simulink model "Controller"  (R2014a)
settings: Solver=FixedStepDiscrete  StartTime=0.0  StopTime=100  FixedStep=0.001  MaxStep=0.01  RelTol=1e-4
InitFcn:
  | Mot_Init
undefined symbols (not defined in the file): Actuator_Length, ControllerRate, Dig_Limit, LowerProtectionFraction, Ratio, SampleSize, UpperProtectionFraction
libraries: simulink x8
settings Model: DSRTSU_INTERNAL_RTI_VER=460  DSRTSU_INTERNAL_RTI_TYPE=rti1006  CovModelRefEnable=off  Creator=jstoddar  LastModifiedBy=uaEcoCar3
settings DataIOCC: SaveFormat=StructureWithTime  SaveOutput=off  SaveTime=off
settings OptimizationCC: ExpressionDepthLimit=2147483647  LifeSpan=1
settings DebuggingCC: UnderspecifiedInitializationDetection=Classic  SolverPrmCheckMsg=none  FcnCallInpInsideContextMsg=EnableAllAsWarning  FrameProcessingCompatibilityMsg=error  StateNameClashWarn=warning
settings HardwareCC: ProdBitPerPointer=64  ProdLargestAtomicFloat=Float  ProdIntDivRoundTo=Zero  ProdEndianess=LittleEndian  ProdHWDeviceType=Specified
settings ModelReferenceCC: PropagateSignalLabelsOutOfModel=on
settings RTWCC: GenCodeOnly=on
settings GRTTargetCC: CombineOutputUpdateFcns=off  GRTInterface=on

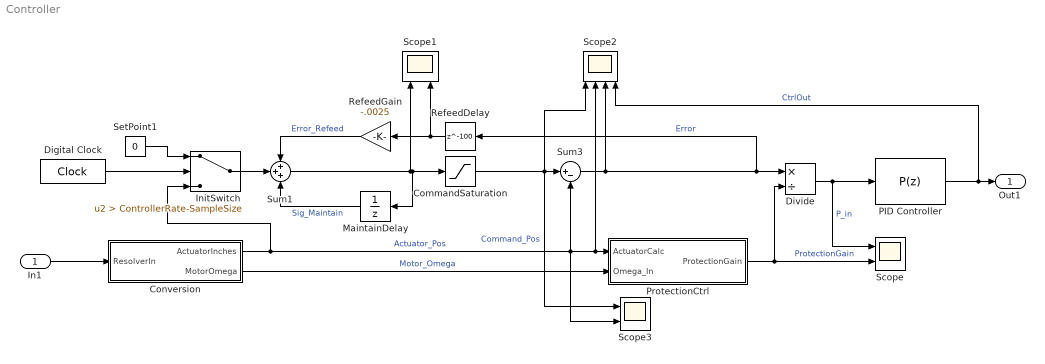
== system Controller ==
  In1 : Inport  OutDataTypeStr=double  PortDimensions=1  SampleTime=[0.001,0]
  CommandSaturation : Saturate  UpperLimit=10  LowerLimit=-10
  Conversion : Subsystem
  Digital Clock : DigitalClock  SampleTime=.001
  Divide : Product  Inputs=*/
  InitSwitch : Switch  Criteria=u2 > Threshold  Threshold=ControllerRate-SampleSize
  MaintainDelay : UnitDelay  SampleTime=-1
  PID Controller : simulink/Continuous/PID Controller  Controller=P  TimeDomain=Discrete-time  SampleTime=-1  IntegratorMethod=Forward Euler  FilterMethod=Forward Euler  Form=Parallel  P=20  I=.1  D=.01  N=4.27601467747136  InitialConditionSource=internal  InitialConditionForIntegrator=0  InitialConditionForFilter=0  ExternalReset=none  LimitOutput=on  UpperSaturationLimit=14  LowerSaturationLimit=-14  LinearizeAsGain=on  AntiWindupMode=none  Kb=1  TrackingMode=off  Kt=1  PParamMin=[]  PParamMax=[]  IParamMin=[]  IParamMax=[]  DParamMin=[]  DParamMax=[]  NParamMin=[]  NParamMax=[]  KbParamMin=[]  KbParamMax=[]  KtParamMin=[]  KtParamMax=[]  POutMin=[]  POutMax=[]  IOutMin=[]  IOutMax=[]  DOutMin=[]  DOutMax=[]  NOutMin=[]  NOutMax=[]  KbOutMin=[]  KbOutMax=[]  KtOutMin=[]  KtOutMax=[]  IntegratorOutMin=[]  IntegratorOutMax=[]  FilterOutMin=[]  FilterOutMax=[]  SumOutMin=[]  SumOutMax=[]  SumI1OutMin=[]  SumI1OutMax=[]  SumI2OutMin=[]  SumI2OutMax=[]  SumI3OutMin=[]  SumI3OutMax=[]  SumDOutMin=[]  SumDOutMax=[]  SaturationOutMin=[]  SaturationOutMax=[]  IntegratorContinuousStateAttributes=''  IntegratorStateMustResolveToSignalObject=off  IntegratorRTWStateStorageClass=Auto  FilterContinuousStateAttributes=''  FilterStateMustResolveToSignalObject=off  FilterRTWStateStorageClass=Auto
  ProtectionCtrl : Subsystem
  RefeedDelay : Delay  DelayLength=100
  RefeedGain : Gain  Gain=-.0025
  Scope : Scope  NumInputPorts=2
      settings: YMin=-0.43586~-5  YMax=1.15954~5
  Scope1 : Scope  NumInputPorts=2
      settings: YMin=-1.25~-0.15204  YMax=11.25~0.01689  SaveName=ScopeData6
  Scope2 : Scope  NumInputPorts=4
      settings: YMin=8.15954~4.375~-0.33852~-12.02188  YMax=10.29522~10.625~0.03761~1.33576  SaveName=ScopeData12
  Scope3 : Scope  NumInputPorts=2
      settings: YMin=-0.72233~-5  YMax=6.50094~5  SaveName=ScopeData7
  SetPoint1 : Constant  Value=0
  Sum1 : Sum  Inputs=+++
  Sum3 : Sum  Inputs=|+-
  Out1 : Outport  OutDataTypeStr=double  PortDimensions=1  SampleTime=[0.001,0]
  wires:
  InitSwitch/1 -> Sum1/2
  CommandSaturation/1 -> Scope2/1, Sum3/1, Scope3/1  "Command_Pos"
  MaintainDelay/1 -> Sum1/3  "Sig_Maintain"
  Sum1/1 -> Scope1/1, MaintainDelay/1, CommandSaturation/1
  RefeedDelay/1 -> Scope1/2, RefeedGain/1
  Digital Clock/1 -> InitSwitch/2
  SetPoint1/1 -> InitSwitch/1
  RefeedGain/1 -> Sum1/1  "Error_Refeed"
  Divide/1 -> PID Controller/1, Scope/1  "P_in"
  Sum3/1 -> Scope2/3, RefeedDelay/1, Divide/1  "Error"
  Conversion/1(ActuatorInches) -> InitSwitch/3, Sum3/2, Scope2/2, ProtectionCtrl/1(ActuatorCalc), Scope3/2  "Actuator_Pos"
  ProtectionCtrl/1(ProtectionGain) -> Scope/2, Divide/2  "ProtectionGain"
  Conversion/2(MotorOmega) -> ProtectionCtrl/2(Omega_In)  "Motor_Omega"
  PID Controller/1 -> Out1/1, Scope2/4  "CtrlOut"
  In1/1 -> Conversion/1(ResolverIn)

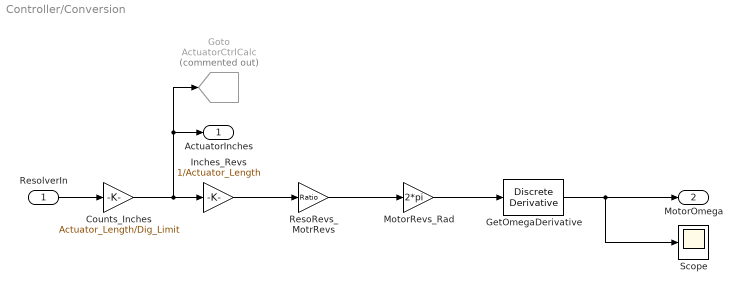
== system Controller/Conversion ==
  ResolverIn : Inport
  Counts_Inches : Gain  Gain=Actuator_Length/Dig_Limit
  GetOmegaDerivative : simulink/Discrete/Discrete Derivative  gainval=1  ICPrevScaledInput=0.0  OutMin=[]  OutMax=[]  OutDataType=fixdt(1, 16)  OutScaling=2^-10  DoSatur=off
  Goto : Goto  Commented=on  GotoTag=ActuatorCtrlCalc  TagVisibility=global
  Inches_Revs : Gain  Gain=1/Actuator_Length
  MotorRevs_Rad : Gain  Gain=2*pi
  ResoRevs_MotrRevs : Gain  Gain=Ratio
  Scope : Scope
      settings: YMin=-19990.6417  YMax=351615.25826  SaveName=ScopeData3
  ActuatorInches : Outport
  MotorOmega : Outport  Port=2
  wires:
  GetOmegaDerivative/1 -> Scope/1, MotorOmega/1
  ResolverIn/1 -> Counts_Inches/1
  MotorRevs_Rad/1 -> GetOmegaDerivative/1
  ResoRevs_MotrRevs/1 -> MotorRevs_Rad/1
  Counts_Inches/1 -> ActuatorInches/1, Goto/1, Inches_Revs/1
  Inches_Revs/1 -> ResoRevs_MotrRevs/1

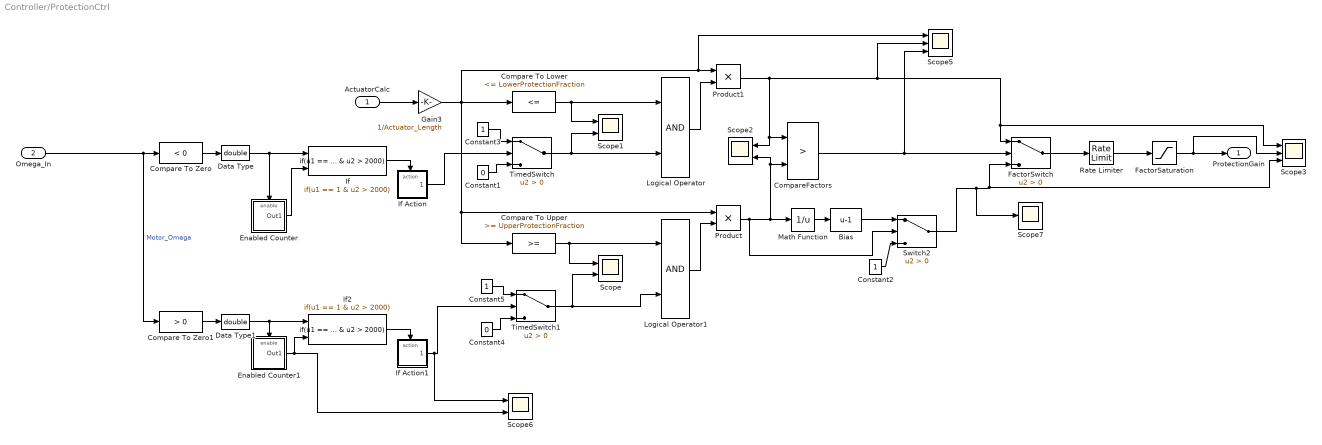
== system Controller/ProtectionCtrl ==
  ActuatorCalc : Inport
  Omega_In : Inport  Port=2
  Bias : Bias  Bias=-1
  Compare To Lower : simulink/Logic and Bit Operations/Compare To Constant  relop=<=  const=LowerProtectionFraction  OutDataTypeStr=boolean
  Compare To Upper : simulink/Logic and Bit Operations/Compare To Constant  relop=>=  const=UpperProtectionFraction  OutDataTypeStr=boolean
  Compare To Zero : simulink/Logic and Bit Operations/Compare To Constant  relop=<  const=0  OutDataTypeStr=boolean
  Compare To Zero1 : simulink/Logic and Bit Operations/Compare To Constant  relop=>  const=0  OutDataTypeStr=boolean
  CompareFactors : RelationalOperator  Operator=>  OutDataTypeStr=boolean  InputSameDT=on
  Constant1 : Constant  Value=0
  Constant2 : Constant
  Constant3 : Constant
  Constant4 : Constant  Value=0
  Constant5 : Constant
  Data Type : DataTypeConversion  OutDataTypeStr=double
  Data Type1 : DataTypeConversion  OutDataTypeStr=double
  Enabled Counter : Subsystem  TreatAsAtomicUnit=on
  Enabled Counter1 : Subsystem  TreatAsAtomicUnit=on
  FactorSaturation : Saturate  UpperLimit=1  LowerLimit=.01
  FactorSwitch : Switch  Criteria=u2 > Threshold
  Gain3 : Gain  Gain=1/Actuator_Length
  If : If  NumInputs=2  IfExpression=u1 == 1 & u2 > 2000  ShowElse=off
  If Action : Subsystem  TreatAsAtomicUnit=on
  If Action1 : Subsystem  TreatAsAtomicUnit=on
  If2 : If  NumInputs=2  IfExpression=u1 == 1 & u2 > 2000  ShowElse=off
  Logical Operator : Logic  AllPortsSameDT=off  OutDataTypeStr=boolean
  Logical Operator1 : Logic  AllPortsSameDT=off  OutDataTypeStr=boolean
  Math Function : Math  Operator=reciprocal  SaturateOnIntegerOverflow=on
  Product : Product
  Product1 : Product
  Rate Limiter : RateLimiter  RisingSlewLimit=1000  FallingSlewLimit=-.3  SampleTimeMode=inherited
  Scope{,1..2,6} (4 alike) : Scope  NumInputPorts=2
      Scope settings: YMin=-0.125~-0.06735  YMax=1.125~1.03444  SaveName=ScopeData2
      Scope1 settings: YMin=-0.125~-0.125  YMax=1.125~1.125  SaveName=ScopeData3
      Scope2 settings: YMin=-1.00000~-0.125  YMax=1.00000~1.125  SaveName=ScopeData4
      Scope6 settings: YMin=-0.125~-11842.875  YMax=1.125~106585.875  SaveName=ScopeData5
  Scope3 : Scope  NumInputPorts=3
      settings: YMin=-1.00000~0.9~0.9  YMax=1.00000~1.1~1.1  SaveName=ScopeData4
  Scope5 : Scope  NumInputPorts=3
      settings: YMin=-0.125~-1.00000~-1.00000  YMax=1.125~1.00000~1.00000  SaveName=ScopeData2
  Scope7 : Scope
      settings: YMin=0.9  YMax=1.1  SaveName=ScopeData4
  Switch2 : Switch  Criteria=u2 > Threshold
  TimedSwitch : Switch  Criteria=u2 > Threshold
  TimedSwitch1 : Switch  Criteria=u2 > Threshold
  ProtectionGain : Outport
  wires:
  Data Type1/1 -> Enabled Counter1/Enable, If2/1
  Data Type/1 -> If/1, Enabled Counter/Enable
  TimedSwitch1/1 -> Logical Operator1/2, Scope/2
  Constant5/1 -> TimedSwitch1/1
  Constant4/1 -> TimedSwitch1/3
  If Action1/1(Out1) -> TimedSwitch1/2, Scope6/1
  If2/1 -> If Action1/Action
  Constant3/1 -> TimedSwitch/1
  Constant1/1 -> TimedSwitch/3
  If Action/1(Out1) -> TimedSwitch/2
  If/1 -> If Action/Action
  Enabled Counter1/1(Out1) -> If2/2, Scope6/2
  Enabled Counter/1(Out1) -> If/2
  Compare To Zero1/1 -> Data Type1/1
  TimedSwitch/1 -> Scope1/2, Logical Operator/2
  Compare To Zero/1 -> Data Type/1
  Rate Limiter/1 -> FactorSaturation/1
  FactorSaturation/1 -> ProtectionGain/1, Scope3/2
  Omega_In/1 -> Compare To Zero/1, Compare To Zero1/1  "Motor_Omega"
  FactorSwitch/1 -> Rate Limiter/1
  Bias/1 -> Switch2/1
  Product1/1 -> Scope3/1, FactorSwitch/1, Scope5/2, CompareFactors/1, Scope2/1
  Product/1 -> Math Function/1, CompareFactors/2, Scope2/2, Switch2/2
  Constant2/1 -> Switch2/3
  CompareFactors/1 -> FactorSwitch/2, Scope5/3
  Switch2/1 -> FactorSwitch/3, Scope3/3, Scope7/1
  Math Function/1 -> Bias/1
  Gain3/1 -> Compare To Upper/1, Product/1, Compare To Lower/1, Product1/1, Scope5/1
  Logical Operator1/1 -> Product/2
  Logical Operator/1 -> Product1/2
  Compare To Upper/1 -> Logical Operator1/1, Scope/1
  Compare To Lower/1 -> Scope1/1, Logical Operator/1
  ActuatorCalc/1 -> Gain3/1

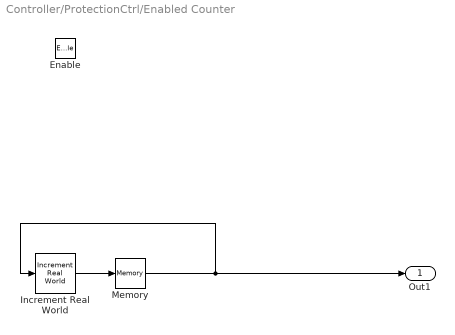
== system Controller/ProtectionCtrl/Enabled Counter ==
  Enable : EnablePort  StatesWhenEnabling=reset
  Increment Real World : simulink/Additional Math & Discrete/Additional Math: Increment - Decrement/Increment Real World  DisableCoverage=on
  Memory : Memory  InheritSampleTime=on  LinearizeAsDelay=on
  Out1 : Outport  OutputWhenDisabled=reset  InitialOutput=0
  wires:
  Memory/1 -> Out1/1, Increment Real World/1
  Increment Real World/1 -> Memory/1

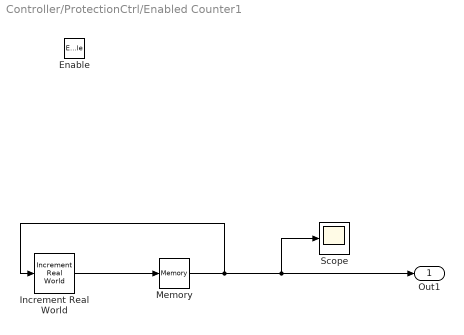
== system Controller/ProtectionCtrl/Enabled Counter1 ==
  Enable : EnablePort  StatesWhenEnabling=reset
  Increment Real World : simulink/Additional Math & Discrete/Additional Math: Increment - Decrement/Increment Real World  DisableCoverage=on
  Memory : Memory  InheritSampleTime=on  LinearizeAsDelay=on
  Scope : Scope
      settings: YMin=-11842.875  YMax=106585.875
  Out1 : Outport  OutputWhenDisabled=reset  InitialOutput=0
  wires:
  Memory/1 -> Scope/1, Out1/1, Increment Real World/1
  Increment Real World/1 -> Memory/1

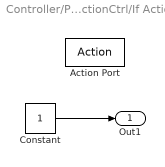
== system Controller/ProtectionCtrl/If Action ==
  Action Port : ActionPort  ActionType=then
  Constant : Constant
  Out1 : Outport  OutputWhenDisabled=reset  InitialOutput=0
  wires:
  Constant/1 -> Out1/1

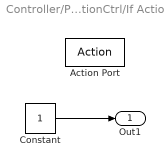
== system Controller/ProtectionCtrl/If Action1 ==
  Action Port : ActionPort  ActionType=then
  Constant : Constant
  Out1 : Outport  OutputWhenDisabled=reset  InitialOutput=0
  wires:
  Constant/1 -> Out1/1
